simulink model "SimplePulseGenerator_4x4_HDL_IQ"  (R2019b)
settings: Solver=FixedStepDiscrete  StartTime=0.0  StopTime=inf  RelTol=1e-3
InitFcn:
  | %axis_example_init
  | nco_setup
  | load('iq_bus_obj.mat')
values from neighbouring files (symbols this model uses):
  Fo = 200.7e6    (= 200700000)    [model_init.m]
  Fs = 1/Ts    (= 512000000)    [model_init.m]
  incrScale = (2^N)/Fs    (= 3.2e-05)    [model_init.m]
  N = 14    [model_init.m]
  PRF_count_period = pspshared.libiio.aximm.write(                    'IPAddress',IPAddr,                    'AddressOffset',hex2dec('130'))    [SimplePulseGenerator_4x4_HDL_IQ_IIO_script.m]    (also in model_init.m = 1280)
  PulseWidth_count_width = PulseWidth*fpga_clk_rate/VectorSamplingFactor    (= 32)    [model_init.m]
libraries: hdlsllib x21, simulink x15, dsphdlsigops x4, simulink_need_slupdate x2, dspsrcs4 x1
(part 2 of 2)

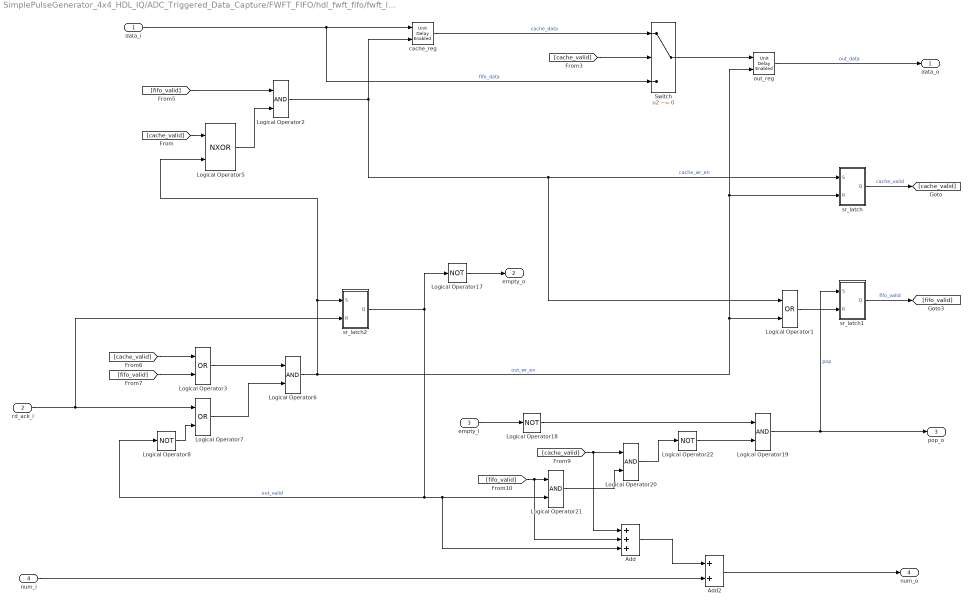
== system SimplePulseGenerator_4x4_HDL_IQ/ADC_Triggered_Data_Capture/FWFT_FIFO/hdl_fwft_fifo/fwft_logic ==
  data_i : Inport
  rd_ack_i : Inport  Port=2
  empty_i : Inport  Port=3
  num_i : Inport  Port=4
  Add : Sum  Inputs=+++  AccumDataTypeStr=fixdt(0,2,0)
  Add2 : Sum  OutDataTypeStr=fixdt(0,FIFO_CNT_BITS,0)
  Logical Operator1 : Logic  Operator=OR  IconShape=distinctive  AllPortsSameDT=off  OutDataTypeStr=boolean
  Logical Operator{8,17..18,22} (4 alike) : Logic  Operator=NOT  IconShape=distinctive  AllPortsSameDT=off  OutDataTypeStr=boolean
  Logical Operator{2,6,19..21} (5 alike) : Logic  IconShape=distinctive  AllPortsSameDT=off  OutDataTypeStr=boolean
  Logical Operator3 : Logic  Operator=OR  IconShape=distinctive  AllPortsSameDT=off  OutDataTypeStr=boolean
  Logical Operator5 : Logic  Operator=NXOR  IconShape=distinctive  AllPortsSameDT=off  OutDataTypeStr=boolean
  Logical Operator7 : Logic  Operator=OR  IconShape=distinctive  AllPortsSameDT=off  OutDataTypeStr=boolean
  Switch : Switch  Criteria=u2 ~= 0
  cache_reg : simulink_need_slupdate/Unit Delay Enabled  vinit=0.0  tsamp=-1
      settings: SourceProductName=Simulink  SourceProductBaseCode=SL
  out_reg : simulink_need_slupdate/Unit Delay Enabled  vinit=0.0  tsamp=-1
      settings: SourceProductName=Simulink  SourceProductBaseCode=SL
  sr_latch : Subsystem
  sr_latch1 : Subsystem
  sr_latch2 : Subsystem
  data_o : Outport  VectorParamsAs1DForOutWhenUnconnected=off
  empty_o : Outport  Port=2  VectorParamsAs1DForOutWhenUnconnected=off
  pop_o : Outport  Port=3  VectorParamsAs1DForOutWhenUnconnected=off
  num_o : Outport  Port=4  VectorParamsAs1DForOutWhenUnconnected=off
  wires:
  empty_i/1 -> Logical Operator18/1
  sr_latch1/1(Q) -> [fifo_valid]  "fifo_valid"
  sr_latch/1(Q) -> [cache_valid]  "cache_valid"
  Switch/1 -> out_reg/1
  data_i/1 -> Switch/3, cache_reg/1  "fifo_data"
  cache_reg/1 -> Switch/1  "cache_data"
  Logical Operator5/1 -> Logical Operator2/2
  Logical Operator6/1 -> Logical Operator5/2, sr_latch2/1(S), out_reg/2, sr_latch/2(R), Logical Operator1/2  "out_wr_en"
  [cache_valid] -> Logical Operator5/1
  [cache_valid] -> Switch/2
  Logical Operator2/1 -> cache_reg/2, Logical Operator1/1, sr_latch/1(S)  "cache_wr_en"
  [fifo_valid] -> Logical Operator2/1
  [cache_valid] -> Logical Operator3/1
  [fifo_valid] -> Logical Operator3/2
  Logical Operator3/1 -> Logical Operator6/1
  Logical Operator7/1 -> Logical Operator6/2
  rd_ack_i/1 -> sr_latch2/2(R), Logical Operator7/1
  sr_latch2/1(Q) -> Logical Operator8/1, Add/3, Logical Operator21/2, Logical Operator17/1  "out_valid"
  Logical Operator8/1 -> Logical Operator7/2
  Logical Operator17/1 -> empty_o/1
  Logical Operator18/1 -> Logical Operator19/1
  Logical Operator21/1 -> Logical Operator20/2
  Logical Operator22/1 -> Logical Operator19/2
  Logical Operator20/1 -> Logical Operator22/1
  Logical Operator19/1 -> pop_o/1, sr_latch1/1(S)  "pop"
  [cache_valid] -> Add/1, Logical Operator20/1
  [fifo_valid] -> Add/2, Logical Operator21/1
  Logical Operator1/1 -> sr_latch1/2(R)
  out_reg/1 -> data_o/1  "out_data"
  num_i/1 -> Add2/2
  Add/1 -> Add2/1
  Add2/1 -> num_o/1

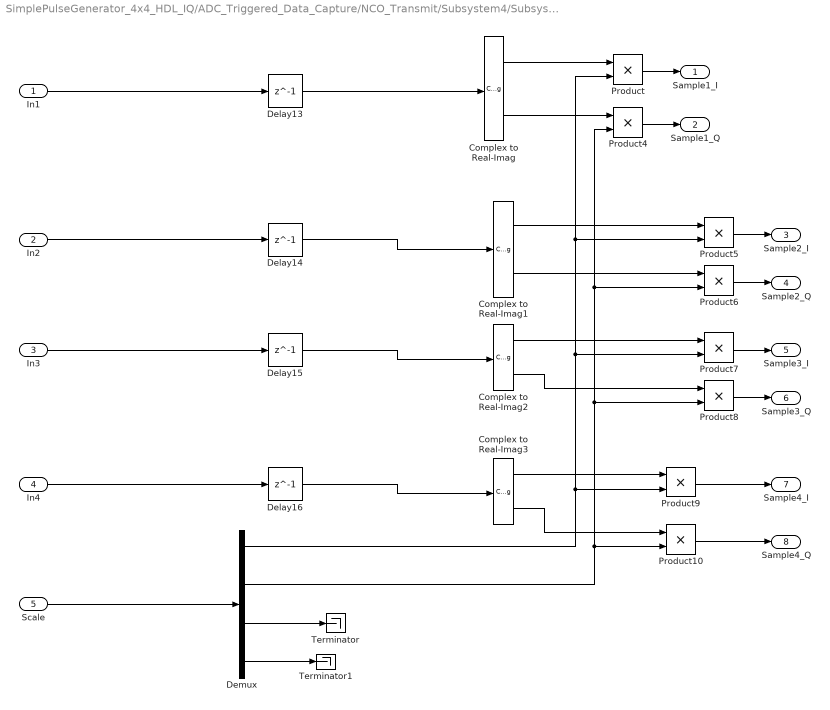
== system SimplePulseGenerator_4x4_HDL_IQ/ADC_Triggered_Data_Capture/NCO_Transmit/Subsystem4/Subsystem ==
  In1 : Inport
  In2 : Inport  Port=2
  In3 : Inport  Port=3
  In4 : Inport  Port=4
  Scale : Inport  Port=5
  Complex to Real-Imag{,1..3} (4 alike) : ComplexToRealImag
  Delay{13..16} (4 alike) : Delay  DelayLength=1
  Demux : Demux
  Product{,4..10} (8 alike) : Product  OutDataTypeStr=Inherit: Same as first input
  Terminator : Terminator
  Terminator1 : Terminator
  Sample1_I : Outport  VectorParamsAs1DForOutWhenUnconnected=off
  Sample1_Q : Outport  Port=2  VectorParamsAs1DForOutWhenUnconnected=off
  Sample2_I : Outport  Port=3  VectorParamsAs1DForOutWhenUnconnected=off
  Sample2_Q : Outport  Port=4  VectorParamsAs1DForOutWhenUnconnected=off
  Sample3_I : Outport  Port=5  VectorParamsAs1DForOutWhenUnconnected=off
  Sample3_Q : Outport  Port=6  VectorParamsAs1DForOutWhenUnconnected=off
  Sample4_I : Outport  Port=7  VectorParamsAs1DForOutWhenUnconnected=off
  Sample4_Q : Outport  Port=8  VectorParamsAs1DForOutWhenUnconnected=off
  wires:
  In1/1 -> Delay13/1
  In3/1 -> Delay15/1
  In2/1 -> Delay14/1
  In4/1 -> Delay16/1
  Delay13/1 -> Complex to Real-Imag/1
  Complex to Real-Imag/1 -> Product/1
  Complex to Real-Imag/2 -> Product4/1
  Delay14/1 -> Complex to Real-Imag1/1
  Delay15/1 -> Complex to Real-Imag2/1
  Delay16/1 -> Complex to Real-Imag3/1
  Product/1 -> Sample1_I/1
  Scale/1 -> Demux/1
  Demux/1 -> Product9/2, Product7/2, Product5/2, Product/2
  Product4/1 -> Sample1_Q/1
  Product5/1 -> Sample2_I/1
  Complex to Real-Imag1/1 -> Product5/1
  Demux/2 -> Product10/2, Product8/2, Product6/2, Product4/2
  Product6/1 -> Sample2_Q/1
  Complex to Real-Imag1/2 -> Product6/1
  Product7/1 -> Sample3_I/1
  Complex to Real-Imag2/1 -> Product7/1
  Complex to Real-Imag2/2 -> Product8/1
  Product8/1 -> Sample3_Q/1
  Complex to Real-Imag3/1 -> Product9/1
  Product9/1 -> Sample4_I/1
  Complex to Real-Imag3/2 -> Product10/1
  Product10/1 -> Sample4_Q/1
  Demux/3 -> Terminator/1
  Demux/4 -> Terminator1/1

== system SimplePulseGenerator_4x4_HDL_IQ/ADC_Triggered_Data_Capture/FWFT_FIFO/hdl_fwft_fifo/fwft_logic/sr_latch ==
  S : Inport
  R : Inport  Port=2
  Logical Operator1 : Logic  IconShape=distinctive  AllPortsSameDT=off  OutDataTypeStr=boolean
  Logical Operator2 : Logic  Operator=NOT  IconShape=distinctive  AllPortsSameDT=off  OutDataTypeStr=boolean
  Logical Operator9 : Logic  Operator=OR  IconShape=distinctive  AllPortsSameDT=off  OutDataTypeStr=boolean
  Unit Delay1 : UnitDelay  SampleTime=-1  HasFrameUpgradeWarning=on
  Q : Outport  VectorParamsAs1DForOutWhenUnconnected=off
  wires:
  S/1 -> Logical Operator9/1
  R/1 -> Logical Operator2/1
  Logical Operator2/1 -> Logical Operator1/1
  Unit Delay1/1 -> Logical Operator1/2, Q/1
  Logical Operator9/1 -> Unit Delay1/1
  Logical Operator1/1 -> Logical Operator9/2

== system SimplePulseGenerator_4x4_HDL_IQ/ADC_Triggered_Data_Capture/FWFT_FIFO/hdl_fwft_fifo/fwft_logic/sr_latch1 ==
  S : Inport
  R : Inport  Port=2
  Logical Operator1 : Logic  IconShape=distinctive  AllPortsSameDT=off  OutDataTypeStr=boolean
  Logical Operator2 : Logic  Operator=NOT  IconShape=distinctive  AllPortsSameDT=off  OutDataTypeStr=boolean
  Logical Operator9 : Logic  Operator=OR  IconShape=distinctive  AllPortsSameDT=off  OutDataTypeStr=boolean
  Unit Delay1 : UnitDelay  SampleTime=-1  HasFrameUpgradeWarning=on
  Q : Outport  VectorParamsAs1DForOutWhenUnconnected=off
  wires:
  Logical Operator1/1 -> Logical Operator9/2
  Logical Operator9/1 -> Unit Delay1/1
  Unit Delay1/1 -> Q/1, Logical Operator1/2
  Logical Operator2/1 -> Logical Operator1/1
  R/1 -> Logical Operator2/1
  S/1 -> Logical Operator9/1

== system SimplePulseGenerator_4x4_HDL_IQ/ADC_Triggered_Data_Capture/FWFT_FIFO/hdl_fwft_fifo/fwft_logic/sr_latch2 ==
  S : Inport
  R : Inport  Port=2
  Logical Operator1 : Logic  IconShape=distinctive  AllPortsSameDT=off  OutDataTypeStr=boolean
  Logical Operator2 : Logic  Operator=NOT  IconShape=distinctive  AllPortsSameDT=off  OutDataTypeStr=boolean
  Logical Operator9 : Logic  Operator=OR  IconShape=distinctive  AllPortsSameDT=off  OutDataTypeStr=boolean
  Unit Delay1 : UnitDelay  SampleTime=-1  HasFrameUpgradeWarning=on
  Q : Outport  VectorParamsAs1DForOutWhenUnconnected=off
  wires:
  S/1 -> Logical Operator9/1
  R/1 -> Logical Operator2/1
  Logical Operator2/1 -> Logical Operator1/1
  Unit Delay1/1 -> Logical Operator1/2, Q/1
  Logical Operator9/1 -> Unit Delay1/1
  Logical Operator1/1 -> Logical Operator9/2

== matlab function SimplePulseGenerator_4x4_HDL_IQ/AXI4Stream_DMA_S2MM/Subsystem2/Subsystem1/MATLAB Function ==
  data: packed_in input; vector_out output; samplesPerClock parameter; complexSamples parameter
function vector_out = fcn(packed_in, samplesPerClock, complexSamples)
%#codegen
%
% unpacks incoming ufixN packed_in into vector_out ([samplesPerClock, 1])
% assumes that samplesPerClock samples are packed into the input
% if complexSamples is true, assumes that I and Q are interleaved so that 
% packed_in is of length samplesPerClock*bitsPerSample*2. Otherwise
% packed_in is of length samplesPerClock*bitsPersample
%
% Greg Ushomirsky, Systems & Technology Research, 2019.
% samplesPerClock = 4;
% complexSamples =true;
bitsPerSample = 16;

if complexSamples
    inputLength = coder.const(samplesPerClock*2);
else
    inputLength = coder.const(samplesPerClock);
end

unpacked_out = zeros(inputLength,1,'like',fi(0,1,bitsPerSample,0));
% elem = int64(0);

% need to unroll this loop at compile time because bitsliceget requires 
% constant inputs 
coder.unroll(); 
for n=1:inputLength
    rightIdx = (n-1)*bitsPerSample + 1;
    leftIdx  = n*bitsPerSample;
    elem =  bitsliceget(packed_in,leftIdx,rightIdx);
    unpacked_out(n) = reinterpretcast(elem, numerictype(1,bitsPerSample,0));
end

if complexSamples
    vector_out = complex(unpacked_out(1:2:end),unpacked_out(2:2:end));
else
    vector_out = unpacked_out;
end
